simulink model "Counter_Task"  (R2021a)
settings: Solver=FixedStepDiscrete  StartTime=0.0  StopTime=10.0  RelTol=1e-3
settings Model: Creator=Mohamed Elomda  LastModifiedBy=Mohamed Elomda
settings OptimizationCC: DefaultParameterBehavior=Inlined  EnhancedBackFolding=on  PassReuseOutputArgsAs=Individual arguments  ZeroExternalMemoryAtStartup=off  ZeroInternalMemoryAtStartup=off  OptimizeBlockOrder=speed  DifferentSizesBufferReuse=on  OptimizationCustomize=off  EfficientTunableParamExpr=on
settings DebuggingCC: UnderspecifiedInitializationDetection=Classic  MergeDetectMultiDrivingBlocksExec=none  ParameterTunabilityLossMsg=error
settings ModelReferenceCC: PropagateSignalLabelsOutOfModel=off
settings SFSimCC: MATLABDynamicMemAlloc=off
settings RTWCC: SystemTargetFile=ert.tlc  GenCodeOnly=on  TemplateMakefile=ert_default_tmf  GenerateReport=on  LaunchReport=on
settings CodeAppCC: ForceParamTrailComments=on  IgnoreCustomStorageClasses=off  OperatorAnnotations=on  SimulinkDataObjDesc=on  SFDataObjDesc=on  InsertBlockDesc=on
settings ERTTargetCC: TargetLangStandard=C99 (ISO)  GenerateSampleERTMain=on  InlinedParameterPlacement=NonHierarchical  ERTCustomFileTemplate=example_file_process.tlc

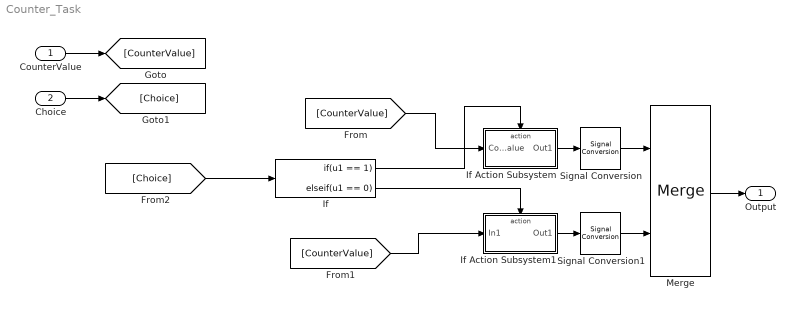
== system Counter_Task ==
  CounterValue : Inport
  Choice : Inport  Port=2
  If : If  IfExpression=u1 == 1  ElseIfExpressions=u1 == 0  ShowElse=off
  If Action Subsystem : Subsystem  TreatAsAtomicUnit=on
  If Action Subsystem1 : Subsystem  TreatAsAtomicUnit=on
  Merge : Merge
  Signal Conversion : SignalConversion  OverrideOpt=off
  Signal Conversion1 : SignalConversion  OverrideOpt=off
  Output : Outport
  wires:
  CounterValue/1 -> [CounterValue]
  If/1 -> If Action Subsystem/Action
  [Choice] -> If/1
  Signal Conversion1/1 -> Merge/2
  Signal Conversion/1 -> Merge/1
  [CounterValue] -> If Action Subsystem/1(CountValue)
  [CounterValue] -> If Action Subsystem1/1(In1)
  If Action Subsystem/1(Out1) -> Signal Conversion/1
  If Action Subsystem1/1(Out1) -> Signal Conversion1/1
  Choice/1 -> [Choice]
  If/2 -> If Action Subsystem1/Action
  Merge/1 -> Output/1

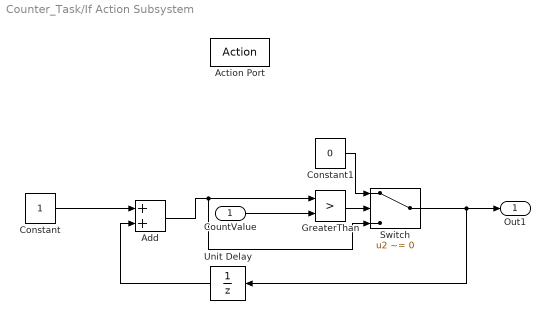
== system Counter_Task/If Action Subsystem ==
  CountValue : Inport
  Action Port : ActionPort  ActionPortLabel=if(u1 == 1)
  Add : Sum
  Constant : Constant
  Constant1 : Constant  Value=0
  GreaterThan : RelationalOperator  Operator=>  OutDataTypeStr=boolean  RndMeth=Simplest
  Switch : Switch  Criteria=u2 ~= 0
  Unit Delay : UnitDelay  InitialCondition=-1  SampleTime=-1  HasFrameUpgradeWarning=on
  Out1 : Outport
  wires:
  Constant/1 -> Add/1
  Unit Delay/1 -> Add/2
  Add/1 -> Switch/3, GreaterThan/1
  GreaterThan/1 -> Switch/2
  Switch/1 -> Unit Delay/1, Out1/1
  Constant1/1 -> Switch/1
  CountValue/1 -> GreaterThan/2

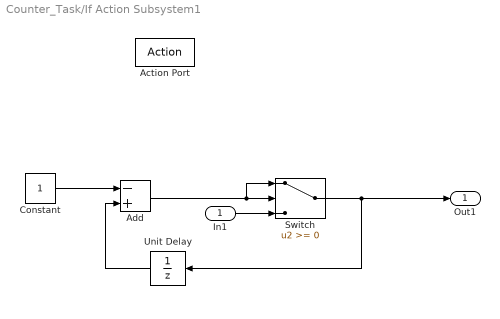
== system Counter_Task/If Action Subsystem1 ==
  In1 : Inport
  Action Port : ActionPort  ActionPortLabel=elseif(u1 == 0)
  Add : Sum  Inputs=-+
  Constant : Constant
  Switch : Switch
  Unit Delay : UnitDelay  SampleTime=-1  HasFrameUpgradeWarning=on
  Out1 : Outport
  wires:
  Constant/1 -> Add/1
  Unit Delay/1 -> Add/2
  Add/1 -> Switch/1, Switch/2
  In1/1 -> Switch/3
  Switch/1 -> Unit Delay/1, Out1/1
